simulink model "DeltaWingPlantADRC"  (R2023b)
settings: Solver=ode45  StartTime=0.0  StopTime=60  MaxStep=0.01  RelTol=1e-3  EnableMultiTasking=on
values from neighbouring files (symbols this model uses):
  betaa0 = 0.4    [int.m]
  betap0 = 0    [int.m]
  Ta = 0.01    [int.m]
libraries: simulink x1
settings Model: Creator=Abel  LastModifiedBy=Abel
settings DataIOCC: LimitDataPoints=on  SaveFormat=Array  SignalLoggingSaveFormat=ModelDataLogs  ReturnWorkspaceOutputs=off
settings OptimizationCC: InitFltsAndDblsToZero=on  LifeSpan=inf
settings DebuggingCC: SaveWithParameterizedLinksMsg=none  UnderspecifiedInitializationDetection=Classic  MergeDetectMultiDrivingBlocksExec=none  SignalResolutionControl=TryResolveAllWithWarning  SolverPrmCheckMsg=warning  MultiTaskDSMMsg=warning  MultiTaskCondExecSysMsg=none  FcnCallInpInsideContextMsg=warning  UnconnectedInputMsg=warning  UnconnectedOutputMsg=warning  UnconnectedLineMsg=warning  SFUnexpectedBacktrackingDiag=warning  SFNoUnconditionalDefaultTransitionDiag=warning  SFExecutionAtInitializationDiag=none  ArithmeticOperatorsInVariantConditions=warning
settings HardwareCC: ProdBitPerPointer=32  ProdBitPerSizeT=32  ProdBitPerPtrDiffT=32  ProdLargestAtomicFloat=None  ProdIntDivRoundTo=Undefined  ProdEndianess=Unspecified  ProdWordSize=32  ProdHWDeviceType=32-bit Generic
settings ModelReferenceCC: PropagateSignalLabelsOutOfModel=off
settings CodeAppCC: StateflowObjectComments=on
settings GRTTargetCC: TargetFcnLib=ansi_tfl_tmw.mat  TargetLangStandard=C89/C90 (ANSI)  CombineOutputUpdateFcns=off  GRTInterface=on
settings ConfigComp: CovMetricSettings=dw  CovSaveCumulativeToWorkspaceVar=on  CovSaveSingleToWorkspaceVar=on

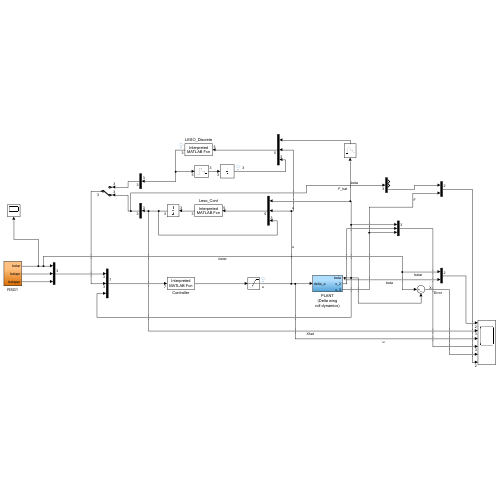
[thumbnail: Simulink's stored preview of the top-level diagram]
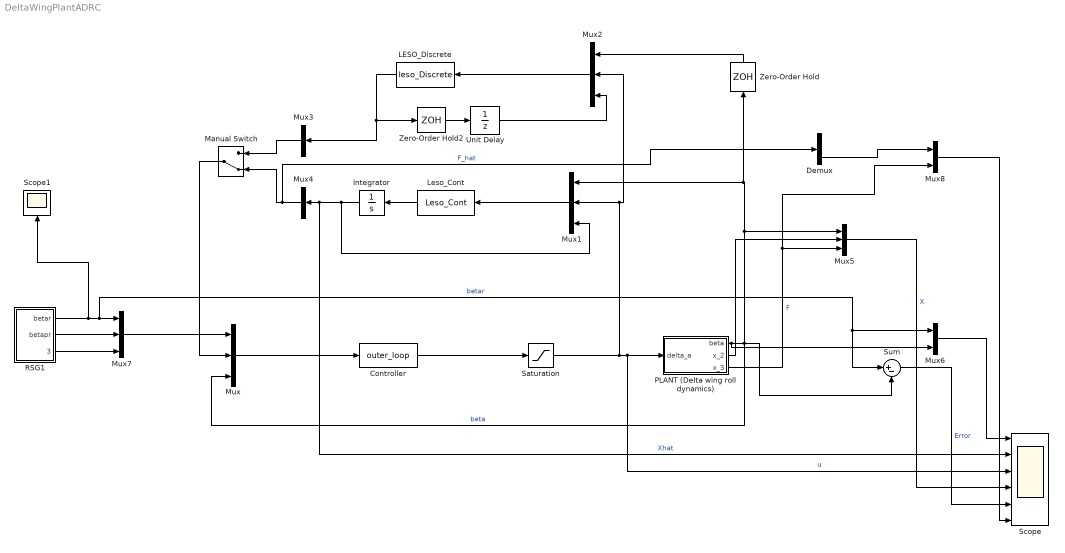
== system DeltaWingPlantADRC ==
  " LESO_Discrete" : MATLABFcn  MATLABFcn=leso_Discrete  OutputDimensions=3
  Controller : MATLABFcn  MATLABFcn=outer_loop  OutputDimensions=1
  Demux : Demux  Outputs=3
  Integrator : Integrator
  Leso_Cont : MATLABFcn  MATLABFcn=Leso_Cont  OutputDimensions=3
  Manual Switch : ManualSwitch  CurrentSetting=0
  Mux : Mux  Inputs=[3 3 1]
  Mux1 : Mux  Inputs=[1 1 3]
  Mux2 : Mux  Inputs=[1 1 3]
  Mux3 : Mux  Inputs=1
  Mux4 : Mux  Inputs=1
  Mux5 : Mux  Inputs=3
  Mux6 : Mux  Inputs=2
  Mux7 : Mux  Inputs=3
  Mux8 : Mux  Inputs=2
  PLANT (Delta wing roll dynamics) : Subsystem
  RSG1 : Subsystem
  Saturation : Saturate  UpperLimit=pi  LowerLimit=-pi
  Scope : Scope  NumInputPorts=6
  Scope1 : Scope
  Sum : Sum  Inputs=|+-
  Unit Delay : UnitDelay  SampleTime=Ta  HasFrameUpgradeWarning=on
  Zero-Order Hold : ZeroOrderHold  SampleTime=Ta
  Zero-Order Hold2 : ZeroOrderHold  SampleTime=Ta
  wires:
  Mux/1 -> Controller/1
  " LESO_Discrete"/1 -> Zero-Order Hold2/1, Mux3/1
  Controller/1 -> Saturation/1
  PLANT (Delta wing roll dynamics)/1(beta) -> Mux6/2, Mux/3, Sum/2, Mux1/1, Zero-Order Hold/1, Mux5/1  "beta"
  Saturation/1 -> Mux2/2, Mux1/2, Scope/3, PLANT (Delta wing roll dynamics)/1(delta_a)  "u"
  Leso_Cont/1 -> Integrator/1
  Mux1/1 -> Leso_Cont/1
  Integrator/1 -> Mux1/3, Scope/2, Mux4/1  "Xhat"
  Mux4/1 -> Demux/1, Manual Switch/2  "F_hat"
  Mux3/1 -> Manual Switch/1
  Manual Switch/1 -> Mux/2
  Sum/1 -> Scope/5  "Error"
  RSG1/1(betar) -> Mux7/1, Sum/1, Mux6/1, Scope1/1  "betar"
  RSG1/2(betapr) -> Mux7/2
  RSG1/3(betappr) -> Mux7/3
  Mux6/1 -> Scope/1
  PLANT (Delta wing roll dynamics)/2(x_2) -> Mux5/2
  PLANT (Delta wing roll dynamics)/3(x_3) -> Mux8/2, Mux5/3  "F"
  Mux2/1 -> " LESO_Discrete"/1
  Unit Delay/1 -> Mux2/3
  Zero-Order Hold2/1 -> Unit Delay/1
  Mux5/1 -> Scope/4  "X"
  Mux8/1 -> Scope/6
  Mux7/1 -> Mux/1
  Zero-Order Hold/1 -> Mux2/1
  Demux/3 -> Mux8/1

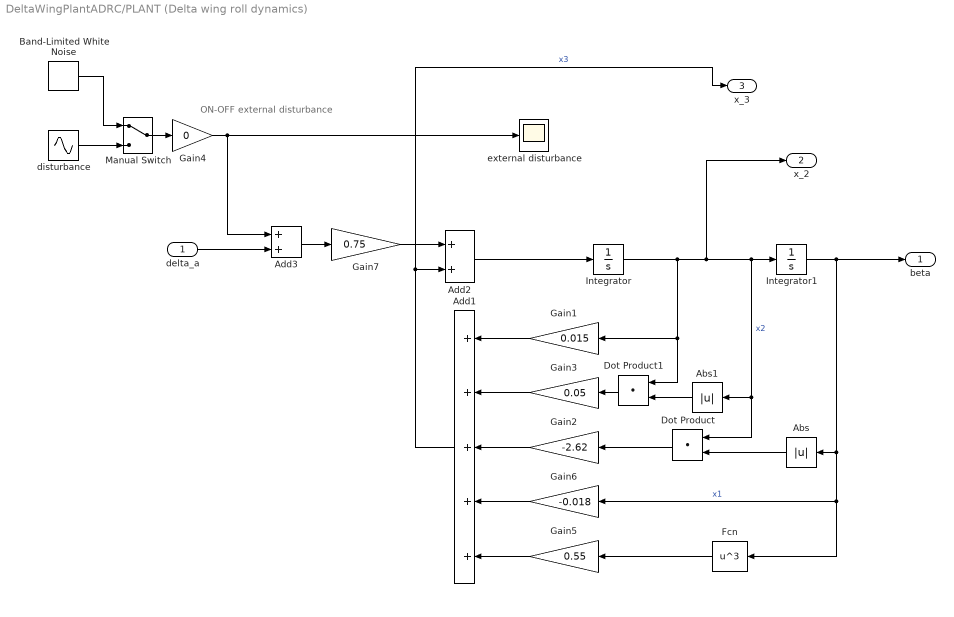
== system DeltaWingPlantADRC/PLANT (Delta wing roll dynamics) ==
  note: ON-OFF external
      | disturbance
  delta_a : Inport
  Abs : Abs  SaturateOnIntegerOverflow=off
  Abs1 : Abs  SaturateOnIntegerOverflow=off
  Add1 : Sum  Inputs=+++++
  Add2 : Sum
  Add3 : Sum
  Band-Limited White Noise : simulink/Sources/Band-Limited White Noise  Cov=[0.1*15]  Ts=15  seed=[23341]
  Dot Product : DotProduct  OutDataTypeStr=Inherit: Inherit via internal rule
  Dot Product1 : DotProduct  OutDataTypeStr=Inherit: Inherit via internal rule
  Fcn : Fcn  Expr=u^3
  Gain1 : Gain  Gain=0.015
  Gain2 : Gain  Gain=-2.62
  Gain3 : Gain  Gain=0.05
  Gain4 : Gain  Gain=0
  Gain5 : Gain  Gain=0.55
  Gain6 : Gain  Gain=-0.018
  Gain7 : Gain  Gain=0.75
  Integrator : Integrator  InitialCondition=betap0  UpperSaturationLimit=pi  LowerSaturationLimit=-pi
  Integrator1 : Integrator  InitialCondition=betaa0
  Manual Switch : ManualSwitch
  disturbance : Sin  Amplitude=1.5  SampleTime=0
  external disturbance : Scope
  beta : Outport
  x_2 : Outport  Port=2
  x_3 : Outport  Port=3
  wires:
  Integrator/1 -> Dot Product1/1, Gain1/1, x_2/1, Integrator1/1, Dot Product/1, Abs1/1  "x2"
  Add2/1 -> Integrator/1
  Manual Switch/1 -> Gain4/1
  Band-Limited White Noise/1 -> Manual Switch/1
  disturbance/1 -> Manual Switch/2
  Integrator1/1 -> beta/1, Gain6/1, Fcn/1, Abs/1  "x1"
  Add1/1 -> x_3/1, Add2/2  "x3"
  Fcn/1 -> Gain5/1
  Dot Product/1 -> Gain2/1
  Abs/1 -> Dot Product/2
  Abs1/1 -> Dot Product1/2
  Dot Product1/1 -> Gain3/1
  Gain1/1 -> Add1/1
  Gain3/1 -> Add1/2
  Gain2/1 -> Add1/3
  Gain6/1 -> Add1/4
  Gain5/1 -> Add1/5
  Gain4/1 -> external disturbance/1, Add3/1
  Add3/1 -> Gain7/1
  delta_a/1 -> Add3/2
  Gain7/1 -> Add2/1

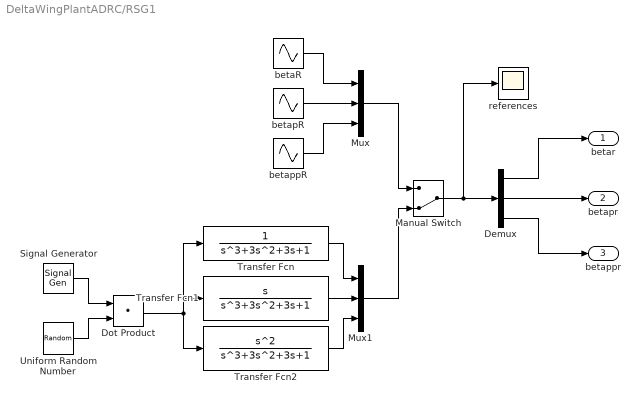
== system DeltaWingPlantADRC/RSG1 ==
  Demux : Demux  Outputs=3
  Dot Product : DotProduct  OutDataTypeStr=Inherit: Inherit via internal rule
  Manual Switch : ManualSwitch  CurrentSetting=0
  Mux : Mux  Inputs=3
  Mux1 : Mux  Inputs=3
  Signal Generator : SignalGenerator  WaveForm=square  Frequency=0.05
  Transfer Fcn : TransferFcn  Denominator=[1 3 3 1]
  Transfer Fcn1 : TransferFcn  Numerator=[1 0]  Denominator=[1 3 3 1]
  Transfer Fcn2 : TransferFcn  Numerator=[1 0 0]  Denominator=[1 3 3 1]
  Uniform Random Number : UniformRandomNumber  Minimum=-0.8*pi/2  Maximum=0.8*pi/2  SampleTime=10
  betaR : Sin  Frequency=0.5  SampleTime=0
  betapR : Sin  Amplitude=0.5  Frequency=0.5  Phase=pi/2  SampleTime=0
  betappR : Sin  Amplitude=-1*0.5*0.5  Frequency=0.5  SampleTime=0
  references : Scope
  betar : Outport
  betapr : Outport  Port=2
  betappr : Outport  Port=3
  wires:
  betaR/1 -> Mux/1
  betapR/1 -> Mux/2
  betappR/1 -> Mux/3
  Mux/1 -> Manual Switch/1
  Mux1/1 -> Manual Switch/2
  Manual Switch/1 -> Demux/1, references/1
  Demux/2 -> betapr/1
  Demux/1 -> betar/1
  Demux/3 -> betappr/1
  Transfer Fcn/1 -> Mux1/1
  Transfer Fcn1/1 -> Mux1/2
  Transfer Fcn2/1 -> Mux1/3
  Signal Generator/1 -> Dot Product/1
  Uniform Random Number/1 -> Dot Product/2
  Dot Product/1 -> Transfer Fcn1/1, Transfer Fcn/1, Transfer Fcn2/1
